simulink library "coeff"  (R2023a)
settings: Solver=VariableStepAuto  StartTime=0.0  StopTime=10.0  RelTol=1e-3
values from neighbouring files (symbols this model uses):
  b = 9.144    [FS.m]
  c = 3.45    [FS.m]
settings Model: Creator=User  LastModifiedBy=User

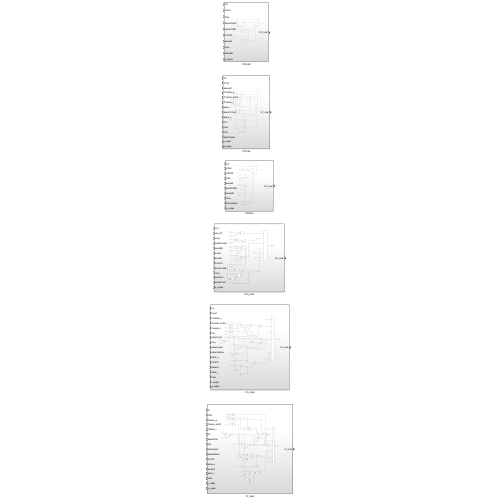
[thumbnail: Simulink's stored preview of the top-level diagram]
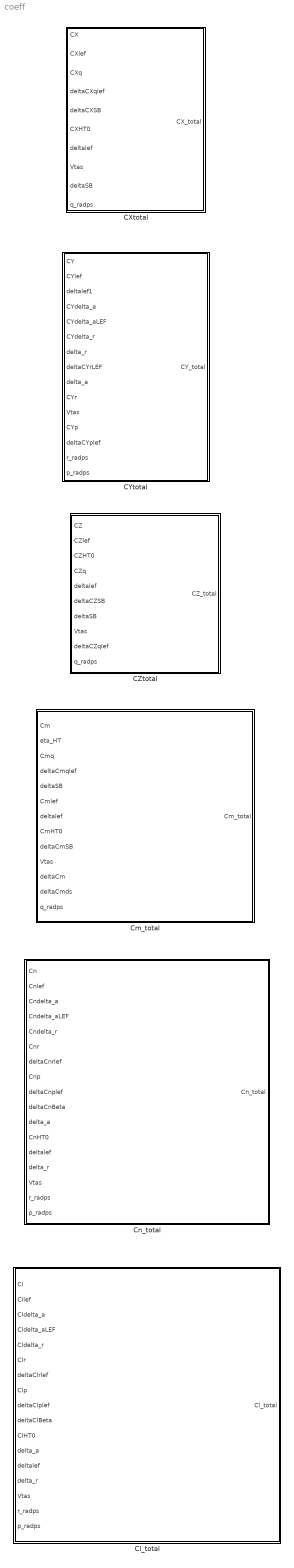
== system coeff ==
  CXtotal : Subsystem
  CYtotal : Subsystem
  CZtotal : Subsystem
  Cl_total : Subsystem
  Cm_total : Subsystem
  Cn_total : Subsystem

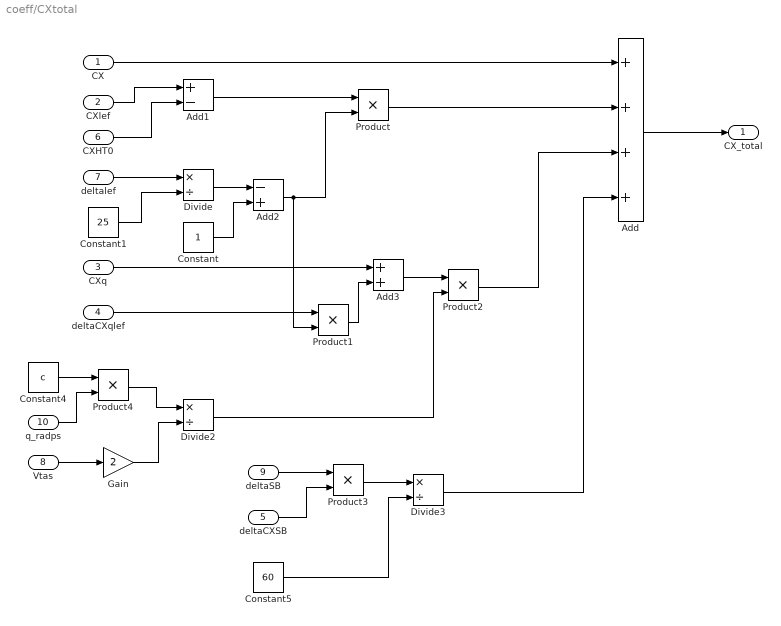
== system coeff/CXtotal ==
  CX : Inport
  CXlef : Inport  Port=2
  CXq : Inport  Port=3
  deltaCXqlef : Inport  Port=4
  deltaCXSB : Inport  Port=5
  CXHT0 : Inport  Port=6
  deltalef : Inport  Port=7
  Vtas : Inport  Port=8
  deltaSB : Inport  Port=9
  q_radps : Inport  Port=10
  Add : Sum  Inputs=++++
  Add1 : Sum  Inputs=+-
  Add2 : Sum  Inputs=-+
  Add3 : Sum
  Constant : Constant
  Constant1 : Constant  Value=25
  Constant4 : Constant  Value=c
  Constant5 : Constant  Value=60
  Divide : Product  Inputs=*/
  Divide2 : Product  Inputs=*/
  Divide3 : Product  Inputs=*/
  Gain : Gain  Gain=2
  Product{,1..4} (5 alike) : Product
  CX_total : Outport
  wires:
  Constant5/1 -> Divide3/2
  Constant1/1 -> Divide/2
  Add/1 -> CX_total/1
  Gain/1 -> Divide2/2
  CX/1 -> Add/1
  Divide/1 -> Add2/1
  CXHT0/1 -> Add1/2
  deltaCXSB/1 -> Product3/2
  Add2/1 -> Product1/2, Product/2
  Product/1 -> Add/2
  Product2/1 -> Add/3
  Product1/1 -> Add3/2
  Vtas/1 -> Gain/1
  Product3/1 -> Divide3/1
  CXq/1 -> Add3/1
  deltalef/1 -> Divide/1
  Constant/1 -> Add2/2
  CXlef/1 -> Add1/1
  Divide2/1 -> Product2/2
  deltaSB/1 -> Product3/1
  Divide3/1 -> Add/4
  Add1/1 -> Product/1
  deltaCXqlef/1 -> Product1/1
  Add3/1 -> Product2/1
  Constant4/1 -> Product4/1
  q_radps/1 -> Product4/2
  Product4/1 -> Divide2/1

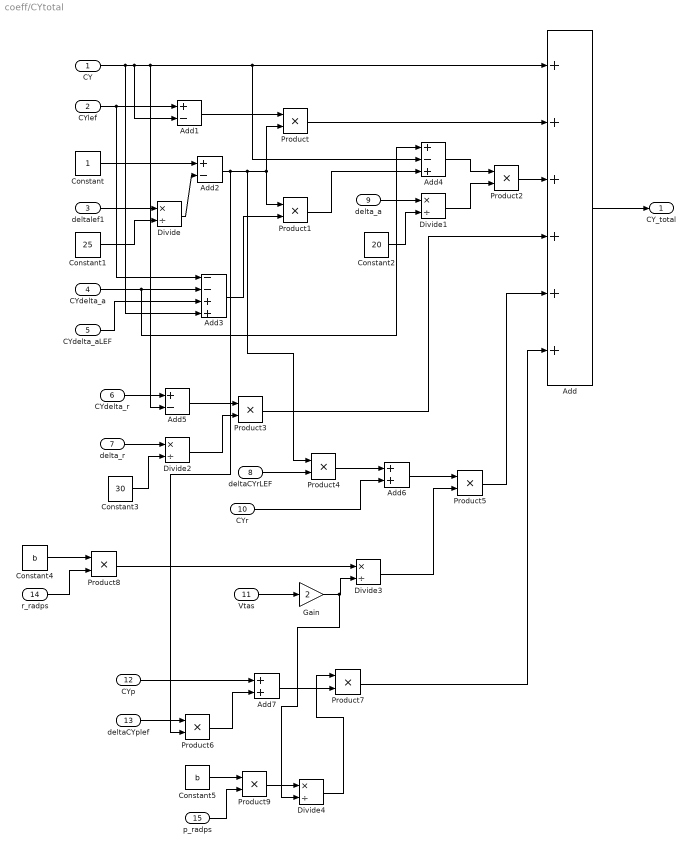
== system coeff/CYtotal ==
  CY : Inport
  CYlef : Inport  Port=2
  deltalef1 : Inport  Port=3
  CYdelta_a : Inport  Port=4
  CYdelta_aLEF : Inport  Port=5
  CYdelta_r : Inport  Port=6
  delta_r : Inport  Port=7
  deltaCYrLEF : Inport  Port=8
  delta_a : Inport  Port=9
  CYr : Inport  Port=10
  Vtas : Inport  Port=11
  CYp : Inport  Port=12
  deltaCYplef : Inport  Port=13
  r_radps : Inport  Port=14
  p_radps : Inport  Port=15
  Add : Sum  Inputs=++++++
  Add1 : Sum  Inputs=+-
  Add2 : Sum  Inputs=+-
  Add3 : Sum  Inputs=--++
  Add4 : Sum  Inputs=+-+
  Add5 : Sum  Inputs=+-
  Add6 : Sum
  Add7 : Sum
  Constant : Constant
  Constant1 : Constant  Value=25
  Constant2 : Constant  Value=20
  Constant3 : Constant  Value=30
  Constant4 : Constant  Value=b
  Constant5 : Constant  Value=b
  Divide{,1..4} (5 alike) : Product  Inputs=*/
  Gain : Gain  Gain=2
  Product{,1..9} (10 alike) : Product
  CY_total : Outport
  wires:
  Add5/1 -> Product3/1
  Gain/1 -> Divide4/2, Divide3/2
  CY/1 -> Add4/2, Add/1, Add5/2, Add1/2, Add3/4
  deltaCYplef/1 -> Product6/1
  Product3/1 -> Add/4
  Divide3/1 -> Product5/2
  CYlef/1 -> Add3/1, Add1/1
  Product7/1 -> Add/6
  CYp/1 -> Add7/1
  Add1/1 -> Product/1
  CYdelta_aLEF/1 -> Add3/3
  Product2/1 -> Add/3
  CYr/1 -> Add6/2
  Add3/1 -> Product1/2
  Add6/1 -> Product5/1
  Add2/1 -> Product6/2, Product4/1, Product1/1, Product/2
  Add4/1 -> Product2/1
  Divide1/1 -> Product2/2
  CYdelta_r/1 -> Add5/1
  CYdelta_a/1 -> Add4/1, Add3/2
  Add7/1 -> Product7/2
  Constant/1 -> Add2/1
  Divide/1 -> Add2/2
  Constant2/1 -> Divide1/2
  Add/1 -> CY_total/1
  Product4/1 -> Add6/1
  Vtas/1 -> Gain/1
  delta_r/1 -> Divide2/1
  deltalef1/1 -> Divide/1
  Constant3/1 -> Divide2/2
  delta_a/1 -> Divide1/1
  Divide2/1 -> Product3/2
  Product1/1 -> Add4/3
  Product6/1 -> Add7/2
  deltaCYrLEF/1 -> Product4/2
  Product/1 -> Add/2
  Constant1/1 -> Divide/2
  Product5/1 -> Add/5
  Constant4/1 -> Product8/1
  r_radps/1 -> Product8/2
  Product8/1 -> Divide3/1
  Constant5/1 -> Product9/1
  p_radps/1 -> Product9/2
  Product9/1 -> Divide4/1
  Divide4/1 -> Product7/1

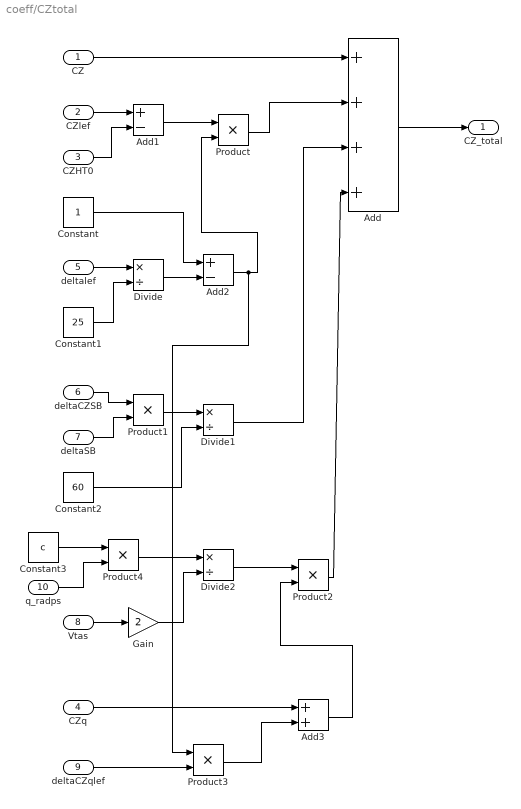
== system coeff/CZtotal ==
  CZ : Inport
  CZlef : Inport  Port=2
  CZHT0 : Inport  Port=3
  CZq : Inport  Port=4
  deltalef : Inport  Port=5
  deltaCZSB : Inport  Port=6
  deltaSB : Inport  Port=7
  Vtas : Inport  Port=8
  deltaCZqlef : Inport  Port=9
  q_radps : Inport  Port=10
  Add : Sum  Inputs=++++
  Add1 : Sum  Inputs=+-
  Add2 : Sum  Inputs=+-
  Add3 : Sum
  Constant : Constant
  Constant1 : Constant  Value=25
  Constant2 : Constant  Value=60
  Constant3 : Constant  Value=c
  Divide : Product  Inputs=*/
  Divide1 : Product  Inputs=*/
  Divide2 : Product  Inputs=*/
  Gain : Gain  Gain=2
  Product{,1..4} (5 alike) : Product
  CZ_total : Outport
  wires:
  CZ/1 -> Add/1
  CZlef/1 -> Add1/1
  CZHT0/1 -> Add1/2
  Add/1 -> CZ_total/1
  deltalef/1 -> Divide/1
  Constant1/1 -> Divide/2
  Divide/1 -> Add2/2
  Constant/1 -> Add2/1
  Add1/1 -> Product/1
  Add2/1 -> Product3/1, Product/2
  Product/1 -> Add/2
  deltaCZSB/1 -> Product1/1
  deltaSB/1 -> Product1/2
  Product1/1 -> Divide1/1
  Constant2/1 -> Divide1/2
  Divide1/1 -> Add/3
  Vtas/1 -> Gain/1
  Gain/1 -> Divide2/2
  Divide2/1 -> Product2/1
  deltaCZqlef/1 -> Product3/2
  CZq/1 -> Add3/1
  Product3/1 -> Add3/2
  Add3/1 -> Product2/2
  Product2/1 -> Add/4
  Product4/1 -> Divide2/1
  Constant3/1 -> Product4/1
  q_radps/1 -> Product4/2

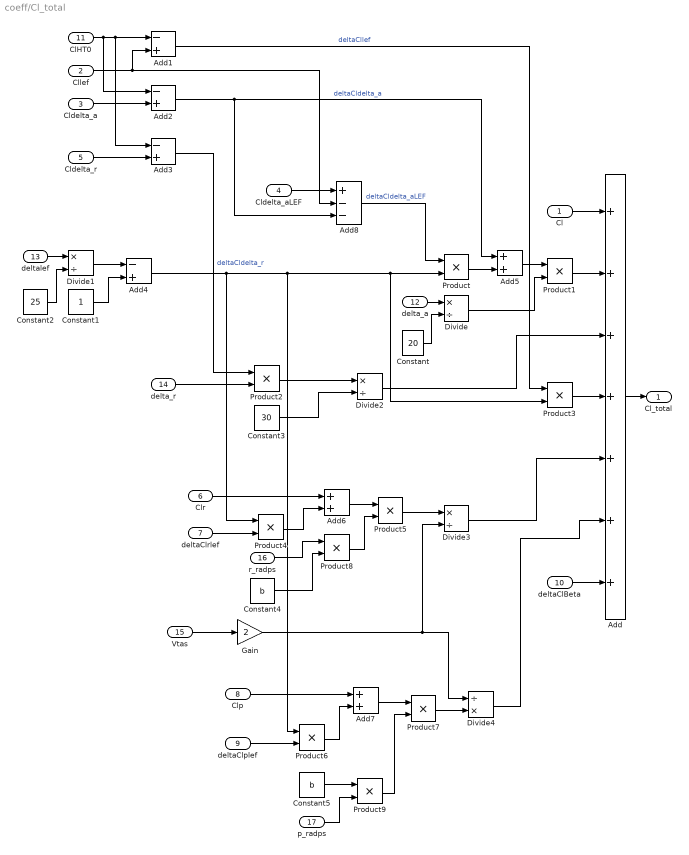
== system coeff/Cl_total ==
  Cl : Inport
  Cllef : Inport  Port=2
  Cldelta_a : Inport  Port=3
  Cldelta_aLEF : Inport  Port=4
  Cldelta_r : Inport  Port=5
  Clr : Inport  Port=6
  deltaClrlef : Inport  Port=7
  Clp : Inport  Port=8
  deltaClplef : Inport  Port=9
  deltaClBeta : Inport  Port=10
  ClHT0 : Inport  Port=11
  delta_a : Inport  Port=12
  deltalef : Inport  Port=13
  delta_r : Inport  Port=14
  Vtas : Inport  Port=15
  r_radps : Inport  Port=16
  p_radps : Inport  Port=17
  Add : Sum  Inputs=+++++++
  Add{1..4} (4 alike) : Sum  Inputs=-+
  Add5 : Sum
  Add6 : Sum
  Add7 : Sum
  Add8 : Sum  Inputs=+--
  Constant : Constant  Value=20
  Constant1 : Constant
  Constant2 : Constant  Value=25
  Constant3 : Constant  Value=30
  Constant4 : Constant  Value=b
  Constant5 : Constant  Value=b
  Divide{,1..3} (4 alike) : Product  Inputs=*/
  Divide4 : Product  Inputs=/*
  Gain : Gain  Gain=2
  Product{,1..9} (10 alike) : Product
  Cl_total : Outport
  wires:
  Cl/1 -> Add/1
  Add/1 -> Cl_total/1
  ClHT0/1 -> Add3/1, Add1/1, Add2/1
  Cllef/1 -> Add8/2, Add1/2
  Cldelta_a/1 -> Add2/2
  Cldelta_r/1 -> Add3/2
  delta_a/1 -> Divide/1
  Constant/1 -> Divide/2
  deltalef/1 -> Divide1/1
  Constant2/1 -> Divide1/2
  Divide1/1 -> Add4/1
  Constant1/1 -> Add4/2
  Add4/1 -> Product/2, Product3/2, Product6/1, Product4/1
  Product/1 -> Add5/2
  Add2/1 -> Add8/3, Add5/1  "deltaCldelta_a"
  Add5/1 -> Product1/1
  Product1/1 -> Add/2
  Divide/1 -> Product1/2
  delta_r/1 -> Product2/2
  Add3/1 -> Product2/1  "deltaCldelta_r"
  Product2/1 -> Divide2/1
  Constant3/1 -> Divide2/2
  Divide2/1 -> Add/3
  Add1/1 -> Product3/1  "deltaCllef"
  Product3/1 -> Add/4
  deltaClBeta/1 -> Add/7
  Clr/1 -> Add6/1
  Product4/1 -> Add6/2
  deltaClrlef/1 -> Product4/2
  Add6/1 -> Product5/1
  Product5/1 -> Divide3/1
  Vtas/1 -> Gain/1
  Divide3/1 -> Add/5
  Product6/1 -> Add7/2
  Add7/1 -> Product7/1
  Clp/1 -> Add7/1
  deltaClplef/1 -> Product6/2
  Divide4/1 -> Add/6
  Product8/1 -> Product5/2
  Constant4/1 -> Product8/2
  r_radps/1 -> Product8/1
  Gain/1 -> Divide3/2, Divide4/1
  Product7/1 -> Divide4/2
  Constant5/1 -> Product9/1
  p_radps/1 -> Product9/2
  Product9/1 -> Product7/2
  Cldelta_aLEF/1 -> Add8/1
  Add8/1 -> Product/1  "deltaCldelta_aLEF"

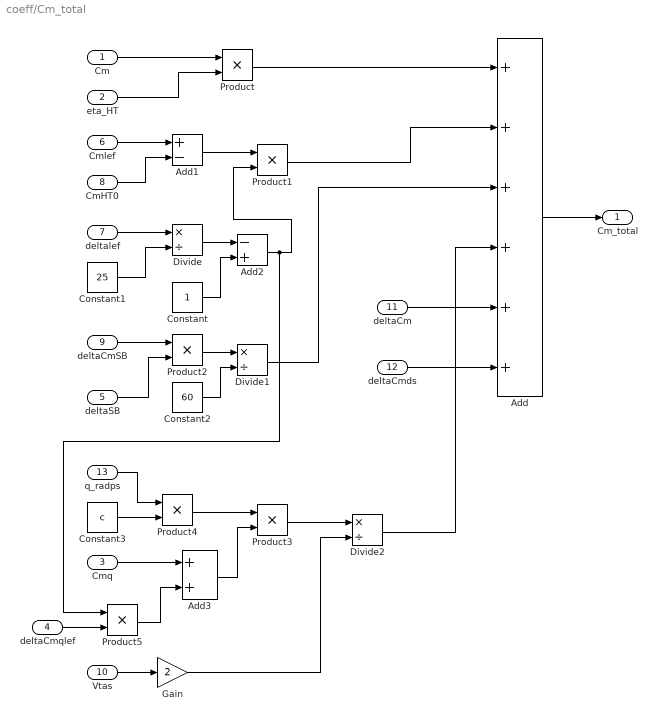
== system coeff/Cm_total ==
  Cm : Inport
  eta_HT : Inport  Port=2
  Cmq : Inport  Port=3
  deltaCmqlef : Inport  Port=4
  deltaSB : Inport  Port=5
  Cmlef : Inport  Port=6
  deltalef : Inport  Port=7
  CmHT0 : Inport  Port=8
  deltaCmSB : Inport  Port=9
  Vtas : Inport  Port=10
  deltaCm : Inport  Port=11
  deltaCmds : Inport  Port=12
  q_radps : Inport  Port=13
  Add : Sum  Inputs=++++++
  Add1 : Sum  Inputs=+-
  Add2 : Sum  Inputs=-+
  Add3 : Sum
  Constant : Constant
  Constant1 : Constant  Value=25
  Constant2 : Constant  Value=60
  Constant3 : Constant  Value=c
  Divide : Product  Inputs=*/
  Divide1 : Product  Inputs=*/
  Divide2 : Product  Inputs=*/
  Gain : Gain  Gain=2
  Product{,1..5} (6 alike) : Product
  Cm_total : Outport
  wires:
  Product/1 -> Add/1
  eta_HT/1 -> Product/2
  Cm/1 -> Product/1
  Add/1 -> Cm_total/1
  Cmlef/1 -> Add1/1
  CmHT0/1 -> Add1/2
  deltalef/1 -> Divide/1
  Constant1/1 -> Divide/2
  Divide/1 -> Add2/1
  Constant/1 -> Add2/2
  Add1/1 -> Product1/1
  Add2/1 -> Product5/1, Product1/2
  Product1/1 -> Add/2
  deltaCmSB/1 -> Product2/1
  deltaSB/1 -> Product2/2
  Product2/1 -> Divide1/1
  Constant2/1 -> Divide1/2
  Divide1/1 -> Add/3
  Add3/1 -> Product3/2
  Vtas/1 -> Gain/1
  Product3/1 -> Divide2/1
  Gain/1 -> Divide2/2
  Divide2/1 -> Add/4
  deltaCm/1 -> Add/5
  deltaCmds/1 -> Add/6
  Constant3/1 -> Product4/2
  q_radps/1 -> Product4/1
  Product4/1 -> Product3/1
  Cmq/1 -> Add3/1
  Product5/1 -> Add3/2
  deltaCmqlef/1 -> Product5/2

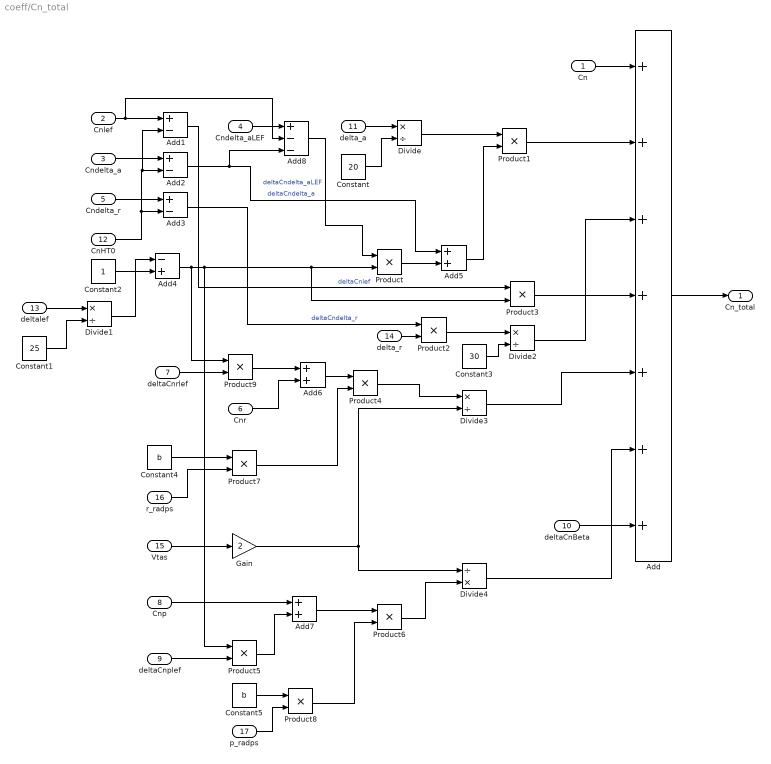
== system coeff/Cn_total ==
  Cn : Inport
  Cnlef : Inport  Port=2
  Cndelta_a : Inport  Port=3
  Cndelta_aLEF : Inport  Port=4
  Cndelta_r : Inport  Port=5
  Cnr : Inport  Port=6
  deltaCnrlef : Inport  Port=7
  Cnp : Inport  Port=8
  deltaCnplef : Inport  Port=9
  deltaCnBeta : Inport  Port=10
  delta_a : Inport  Port=11
  CnHT0 : Inport  Port=12
  deltalef : Inport  Port=13
  delta_r : Inport  Port=14
  Vtas : Inport  Port=15
  r_radps : Inport  Port=16
  p_radps : Inport  Port=17
  Add : Sum  Inputs=+++++++
  Add1 : Sum  Inputs=+-
  Add2 : Sum  Inputs=+-
  Add3 : Sum  Inputs=+-
  Add4 : Sum  Inputs=-+
  Add5 : Sum
  Add6 : Sum
  Add7 : Sum
  Add8 : Sum  Inputs=+--
  Constant : Constant  Value=20
  Constant1 : Constant  Value=25
  Constant2 : Constant
  Constant3 : Constant  Value=30
  Constant4 : Constant  Value=b
  Constant5 : Constant  Value=b
  Divide{,1..3} (4 alike) : Product  Inputs=*/
  Divide4 : Product  Inputs=/*
  Gain : Gain  Gain=2
  Product{,1..9} (10 alike) : Product
  Cn_total : Outport
  wires:
  Add/1 -> Cn_total/1
  Cn/1 -> Add/1
  delta_a/1 -> Divide/1
  Constant/1 -> Divide/2
  Cnlef/1 -> Add8/2, Add1/1
  Cndelta_a/1 -> Add2/1
  Cndelta_r/1 -> Add3/1
  CnHT0/1 -> Add1/2, Add2/2, Add3/2
  Constant1/1 -> Divide1/2
  deltalef/1 -> Divide1/1
  Add4/1 -> Product9/1, Product5/1, Product3/2, Product/2
  Product/1 -> Add5/2
  Add2/1 -> Add8/3, Add5/1  "deltaCndelta_a"
  Divide/1 -> Product1/1
  Add5/1 -> Product1/2
  Product1/1 -> Add/2
  Add3/1 -> Product2/1  "deltaCndelta_r"
  delta_r/1 -> Product2/2
  Product2/1 -> Divide2/1
  Constant3/1 -> Divide2/2
  Divide2/1 -> Add/3
  Add1/1 -> Product3/1  "deltaCnlef"
  Product3/1 -> Add/4
  Add6/1 -> Product4/1
  Product4/1 -> Divide3/1
  Vtas/1 -> Gain/1
  Gain/1 -> Divide4/1, Divide3/2
  Divide3/1 -> Add/5
  deltaCnBeta/1 -> Add/7
  Cnp/1 -> Add7/1
  deltaCnplef/1 -> Product5/2
  Product5/1 -> Add7/2
  Add7/1 -> Product6/1
  Divide4/1 -> Add/6
  Cnr/1 -> Add6/2
  Product7/1 -> Product4/2
  Constant4/1 -> Product7/1
  r_radps/1 -> Product7/2
  Constant5/1 -> Product8/1
  p_radps/1 -> Product8/2
  Product8/1 -> Product6/2
  Constant2/1 -> Add4/2
  Divide1/1 -> Add4/1
  Product9/1 -> Add6/1
  deltaCnrlef/1 -> Product9/2
  Add8/1 -> Product/1  "deltaCndelta_aLEF"
  Cndelta_aLEF/1 -> Add8/1
  Product6/1 -> Divide4/2
